simulink library "create_THB"  (R2016b)
settings: Solver=ode45  StartTime=0.0  StopTime=10.0  RelTol=1e-3  EnableMultiTasking=on
undefined symbols (not defined in the file): Water
libraries: carnot x1
settings Model: Creator=lena.frank  LastModifiedBy=drhf
settings DataIOCC: LimitDataPoints=on  SaveFormat=Array  SignalLoggingSaveFormat=ModelDataLogs
settings OptimizationCC: ExpressionDepthLimit=2147483647  LifeSpan=inf
settings DebuggingCC: UnderspecifiedInitializationDetection=Classic  MergeDetectMultiDrivingBlocksExec=none  SolverPrmCheckMsg=warning  FcnCallInpInsideContextMsg=warning  StateNameClashWarn=warning  SFUnexpectedBacktrackingDiag=warning  SFNoUnconditionalDefaultTransitionDiag=warning  SFExecutionAtInitializationDiag=none
settings HardwareCC: ProdBitPerPointer=32  ProdBitPerSizeT=32  ProdBitPerPtrDiffT=32  ProdLargestAtomicFloat=None  ProdIntDivRoundTo=Undefined  ProdEndianess=Unspecified  ProdWordSize=32  ProdHWDeviceType=32-bit Generic
settings ModelReferenceCC: PropagateSignalLabelsOutOfModel=off
settings GRTTargetCC: TargetLangStandard=C89/C90 (ANSI)  GeneratePreprocessorConditionals=Disable all  CombineOutputUpdateFcns=off  GRTInterface=on
settings ConfigComp: CovMetricSettings=dw  CovHtmlReporting=on  CovSaveCumulativeToWorkspaceVar=on  CovSaveSingleToWorkspaceVar=on  CovExternalEMLEnable=off

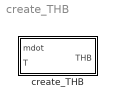
== system create_THB ==
  create_THB : Subsystem  mask(create THB){p=1e5, fluid=Water, mix=0, mix2=0, mix3=0, dia=0, hgt=0, mID=No Pressure Drop}
      mask prompts: p "pressure [Pa]"; mix "fluid mixture [0..1]"; mix2 "fluid mixture 2 [0..1]"; mix3 "fluid mixture 3 [0..1]"; dia "diameter [m]"; hgt "Geodetic height in m"; mID "ID (for pressure drop calculation)"
      mask help: Block to create a THB with the variable input T and mdot. The other value can be set as constants in the mask.
      mask init:
      | mix = min(1, max(0, mix));
      | dia = max(dia, 0.001);
      | ID = (mID-1)*10000+1;
      mask Help: web(fullfile(path_carnot('help'),'createTHB.html'),'-helpbrowser')
      mask TypeOptions p: basic_create_THB/p
      mask TypeOptions fluid: basic_create_THB/fluid
      mask TypeOptions mix: basic_create_THB/mix
      mask TypeOptions mix2: basic_create_THB/mix2
      mask TypeOptions mix3: basic_create_THB/mix3
      mask TypeOptions dia: basic_create_THB/dia
      mask TypeOptions hgt: basic_create_THB/hgt
      mask TypeOptions mID: basic_create_THB/mID

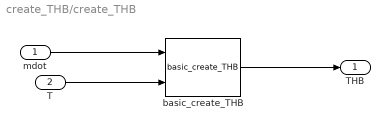
== system create_THB/create_THB ==
  mdot : Inport
  T : Inport  Port=2
  basic_create_THB : carnot/Basic/Hydraulics/basic_create_THB  p=p  fluid=Water  mix=mix  mix2=mix2  mix3=mix3  dia=dia  hgt=hgt  mID=No Pressure Drop
  THB : Outport
  wires:
  T/1 -> basic_create_THB/2
  basic_create_THB/1 -> THB/1
  mdot/1 -> basic_create_THB/1
